simulink model "Processo_PI"  (R2016a)
settings: Solver=VariableStepAuto  StartTime=0.0  StopTime=20  RelTol=1e-3
settings Model: Creator=mende  LastModifiedBy=mende

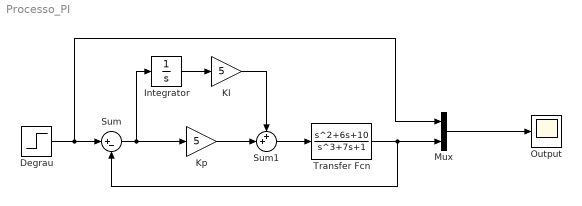
== system Processo_PI ==
  Degrau : Step  SampleTime=0
  Integrator : Integrator
  KI : Gain  Gain=5
  Kp : Gain  Gain=5
  Mux : Mux  Inputs=2
  Output : Scope
  Sum : Sum  Inputs=|+-
  Sum1 : Sum  Inputs=++|
  Transfer Fcn : TransferFcn  Numerator=[1,6,10]  Denominator=[1,0,7,1]
  wires:
  Degrau/1 -> Mux/1, Sum/1
  Transfer Fcn/1 -> Mux/2, Sum/2
  Sum/1 -> Integrator/1, Kp/1
  Mux/1 -> Output/1
  Integrator/1 -> KI/1
  Sum1/1 -> Transfer Fcn/1
  Kp/1 -> Sum1/2
  KI/1 -> Sum1/1
